simulink model "Three_torques_inputs"  (R2014b)
settings: Solver=ode45  SolverMode=SingleTasking  StartTime=0.0  StopTime=10.0  MaxStep=0.01  RelTol=1e-3
values from neighbouring files (symbols this model uses):
  A = eval(As)    [Three_torque_input.m]    (also in plotting_script.m)
  B = eval(Bs)    [Three_torque_input.m]    (also in plotting_script.m)
  Kr = -inv(Cc*inv(Aa-Bb*K)*Bb)    [Three_torque_input.m]    (also in plotting_script.m = (-inv(Cs*inv(Aa-Bb*K)*Bb)))
undefined symbols (not defined in the file or in its folder): sigbuilder_block
settings Model: CovSFcnEnable=on  Creator=Jaby  LastModifiedBy=danielpihlquist
settings OptimizationCC: BlockReduction=off  BooleanDataType=off  UseDivisionForNetSlopeComputation=off  SimCompilerOptimization=off
settings DebuggingCC: SaveWithParameterizedLinksMsg=none  UnderspecifiedInitializationDetection=Classic  MergeDetectMultiDrivingBlocksExec=none  SignalResolutionControl=TryResolveAllWithWarning  SolverPrmCheckMsg=none  FrameProcessingCompatibilityMsg=error
settings HardwareCC: TargetUnknown=on
settings RTWCC: RTWCompilerOptimization=off

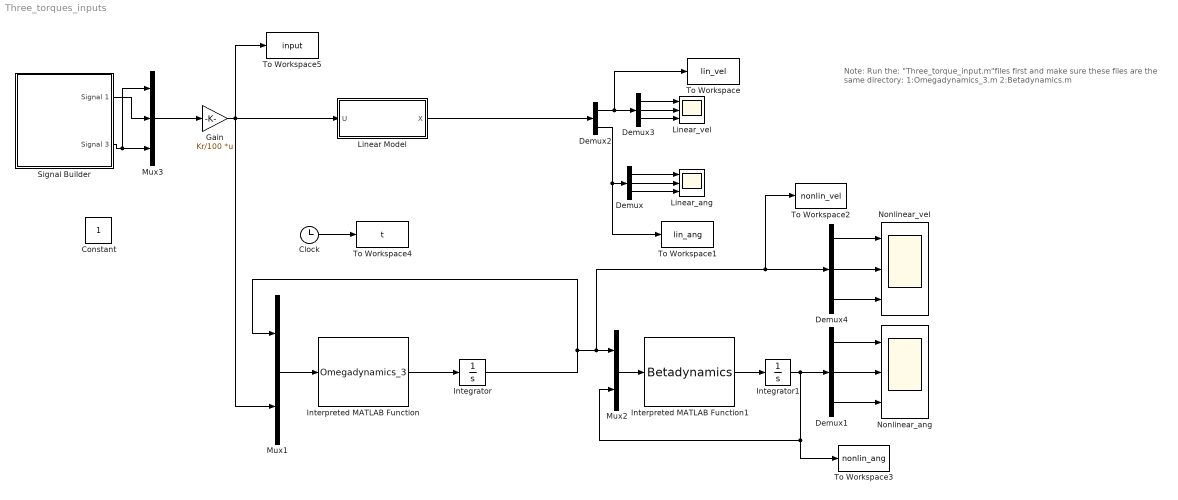
== system Three_torques_inputs ==
  note: Note:
      | Run the: "Three_torque_input.m"files first
      | and make sure these files are the same directory:
      | 1:Omegadynamics_3.m
      | 2:Betadynamics.m
  Clock : Clock
  Constant : Constant
  Demux{,1,3..4} (4 alike) : Demux  Outputs=3
  Demux2 : Demux  Outputs=2
  Gain : Gain  Gain=Kr/100  Multiplication=Matrix(K*u)
  Integrator : Integrator  InitialCondition=[0 0 0]'
  Integrator1 : Integrator  InitialCondition=[0 0 0]'
  Interpreted MATLAB Function : MATLABFcn  MATLABFcn=Omegadynamics_3  Output1D=off
  Interpreted MATLAB Function1 : MATLABFcn  MATLABFcn=Betadynamics  Output1D=off
  "Linear Model " : Subsystem
  Linear_ang : Scope  NumInputPorts=3
      settings: TimeRange=20  YMin=0.00274~-3.07e-14~8.3e-31  YMax=0.00278~-3.025e-14~8.43e-31
  Linear_vel : Scope  NumInputPorts=3
      settings: TimeRange=20  YMin=0~0~-1  YMax=2e+07~7000~1  SaveName=ScopeData2
  Mux1 : Mux  Inputs=2
  Mux2 : Mux  Inputs=2
  Mux3 : Mux  Inputs=3
  Nonlinear_ang : Scope  NumInputPorts=3
      settings: YMin=-5~-5~-5  YMax=5~5~5
  Nonlinear_vel : Scope  NumInputPorts=3
      settings: TimeRange=10  YMin=-5~-5~-5  YMax=5~5~5  SaveName=ScopeData3
  Signal Builder : Subsystem  Tag=STV Subsys  LoadFcn=sigbuilder_block('load');  StartFcn=sigbuilder_block('start');  StopFcn=sigbuilder_block('stop');  ClipboardFcn=sigbuilder_block('clipboard');  mask(Sigbuilder block){}
      mask help: Simulink:masks:SigbuilderBlock_MD
      mask init:
      | if ~strcmp(get_param(bdroot(gcbh),'SimulationStatus'),'stopped') tuvar = sigbuilder_block('maskInit'); end
      settings: CopyFcn=sigbuilder_block('copy');  DeleteFcn=sigbuilder_block('delete');  ModelCloseFcn=sigbuilder_block('modelClose');  PreSaveFcn=sigbuilder_block('preSave');  PauseFcn=sigbuilder_block('pause');  ContinueFcn=sigbuilder_block('continue');  NameChangeFcn=sigbuilder_block('namechange');  OpenFcn=sigbuilder_block('open',[437.6 199.2 550.4 400 ]);  CloseFcn=sigbuilder_block('close');
      mask Display: plot(0, 0, 100, 100,[2, 2, 32, 32, 2], [68, 8, 8, 68, 68],[32, 2], [38, 38], [32, 19, 2],[53, 60, 44], [32, 17, 17, 2],[16, 16, 31, 31]);txt = getActiveGroup(gcbh);text(2, 100, txt,'verticalAlignment', 'top');
  To Workspace : ToWorkspace  VariableName=lin_vel  SampleTime=-1
  To Workspace1 : ToWorkspace  VariableName=lin_ang  SampleTime=-1
  To Workspace2 : ToWorkspace  VariableName=nonlin_vel  SampleTime=-1
  To Workspace3 : ToWorkspace  VariableName=nonlin_ang  SampleTime=-1
  To Workspace4 : ToWorkspace  VariableName=t  SampleTime=-1
  To Workspace5 : ToWorkspace  VariableName=input  SampleTime=-1
  wires:
  "Linear Model "/1(X) -> Demux2/1
  Demux/1 -> Linear_ang/1
  Demux/2 -> Linear_ang/2
  Demux/3 -> Linear_ang/3
  Mux1/1 -> Interpreted MATLAB Function/1
  Interpreted MATLAB Function/1 -> Integrator/1
  Interpreted MATLAB Function1/1 -> Integrator1/1
  Demux1/2 -> Nonlinear_ang/2
  Integrator1/1 -> Demux1/1, To Workspace3/1, Mux2/2
  Demux1/3 -> Nonlinear_ang/3
  Demux1/1 -> Nonlinear_ang/1
  Mux2/1 -> Interpreted MATLAB Function1/1
  Demux2/2 -> To Workspace1/1, Demux/1
  Demux3/1 -> Linear_vel/1
  Demux3/2 -> Linear_vel/2
  Demux3/3 -> Linear_vel/3
  Demux2/1 -> To Workspace/1, Demux3/1
  Mux3/1 -> Gain/1
  Demux4/2 -> Nonlinear_vel/2
  Demux4/3 -> Nonlinear_vel/3
  Demux4/1 -> Nonlinear_vel/1
  Integrator/1 -> To Workspace2/1, Demux4/1, Mux2/1, Mux1/1
  Clock/1 -> To Workspace4/1
  Signal Builder/2(Signal 3) -> Mux3/1, Mux3/3
  Gain/1 -> Mux1/2, To Workspace5/1, "Linear Model "/1(U)
  Signal Builder/1(Signal 1) -> Mux3/2

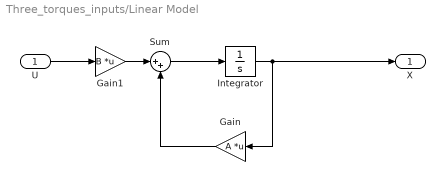
== system Three_torques_inputs/Linear Model  ==
  U : Inport
  Gain : Gain  Gain=A  Multiplication=Matrix(K*u)
  Gain1 : Gain  Gain=B  Multiplication=Matrix(K*u)
  Integrator : Integrator
  Sum : Sum  Inputs=|++
  X : Outport
  wires:
  Integrator/1 -> X/1, Gain/1
  U/1 -> Gain1/1
  Gain1/1 -> Sum/1
  Sum/1 -> Integrator/1
  Gain/1 -> Sum/2

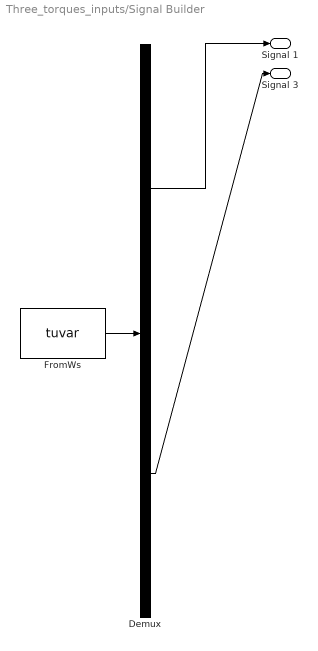
== system Three_torques_inputs/Signal Builder ==
  Demux : Demux  Tag=STV Demux  Outputs=2
  FromWs : FromWorkspace  Tag=STV FromWs  VariableName=tuvar  SampleTime=0
      SigBuilderData=|
      | common.afterFinalStr = 'Extrapolate'
      | common.sampleTime = 0
      | dataSet.timeRange = [0 20]
      | dataSet.name = 'Group 1'
      | sbobj.Groups.Name = 'Group 1'
      | sbobj.Groups.Signals(1).Name = 'Signal 1'
      | sbobj.Groups.Signals(1).XData = [0 1 1 1.55 1.55 20]
      | sbobj.Groups.Signals(1).YData = [0 0 1 1 0 0]
      | sbobj.Groups.Signals(2).Name = 'Signal 3'
      | sbobj.Groups.Signals(2).XData = [0 11.15 11.15 11.85 11.85 20]
      | sbobj.Groups.Signals(2).YData = [0 0 1 1 0 0]
      | sbobj.Groups.TimeRange = [0 20]
  Signal 1 : Outport  Tag=STV Outport
  Signal 3 : Outport  Tag=STV Outport  Port=2
  wires:
  Demux/1 -> Signal 1/1
  FromWs/1 -> Demux/1
  Demux/2 -> Signal 3/1
